simulink model "rtwdemo_structparam"  (Simulink 7.1)
settings: Solver=FixedStepDiscrete  StartTime=0.0  StopTime=10.0  RelTol=1e-3
PostLoadFcn:
  | load structparams.mat;
undefined symbols (not defined in the file or in its folder): p_1, p_2, p_3
settings Model: Creator=ajayaram  LastModifiedBy=ajayaram
settings OptimizationCC: InlineParams=on  OptimizeModelRefInitCode=on  LifeSpan=1
settings RTWCC: SystemTargetFile=ert.tlc  TemplateMakefile=ert_default_tmf  Description=Real-Time Workshop Embedded Coder (no auto configuration)  GenerateReport=on  ProcessScript=ert_make_rtw_hook  IncludeHyperlinkInReport=on  LaunchReport=on
settings CodeAppCC: IgnoreCustomStorageClasses=off
settings ERTTargetCC: GenerateSampleERTMain=on  InlinedParameterPlacement=NonHierarchical  ERTCustomFileTemplate=example_file_process.tlc

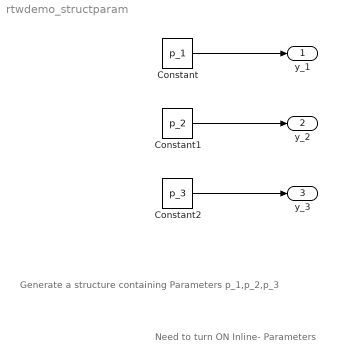
== system rtwdemo_structparam ==
  note: Need to turn ON Inline- Parameters
  note: Generate a structure
      | containing Parameters
      | p_1,p_2,p_3
  Constant : Constant  Value=p_1  OutDataType=sfix(16)  OutScaling=2^0
  Constant1 : Constant  Value=p_2  OutDataType=sfix(16)  OutScaling=2^0
  Constant2 : Constant  Value=p_3  OutDataType=sfix(16)  OutScaling=2^0
  y_1 : Outport  OutDataType=sfix(16)  OutScaling=2^0
  y_2 : Outport  Port=2  OutDataType=sfix(16)  OutScaling=2^0
  y_3 : Outport  Port=3  OutDataType=sfix(16)  OutScaling=2^0
  wires:
  Constant/1 -> y_1/1
  Constant1/1 -> y_2/1
  Constant2/1 -> y_3/1
